simulink model "simulink_model_S"  (R2022a)
settings: Solver=VariableStepAuto  StartTime=0.0  StopTime=100  RelTol=1e-3
values from neighbouring files (symbols this model uses):
  b1 = 8    [Simulink_model_M.m]    (also in Stavovy_model_G1_M.m; Stavovy_model_G2_M.m)
  b2 = 1.6    [Simulink_model_M.m]    (also in Stavovy_model_G1_M.m; Stavovy_model_G2_M.m; Vysetrenie_vplyvu_zmeny_parametrov_G3.m = double(b2))
  F2 = 0    [Simulink_model_M.m]    (also in Stavovy_model_G1_M.m; Stavovy_model_G2_M.m)
  k1 = 400    [Simulink_model_M.m]    (also in Stavovy_model_G1_M.m; Stavovy_model_G2_M.m)
  k2 = 80    [Simulink_model_M.m]    (also in Stavovy_model_G1_M.m; Stavovy_model_G2_M.m)
  m1 = 0.5    [Simulink_model_M.m]    (also in Stavovy_model_G1_M.m; Stavovy_model_G2_M.m)
  m2 = 0.1    [Simulink_model_M.m]    (also in Stavovy_model_G1_M.m; Stavovy_model_G2_M.m)
settings Model: Creator=Ivan  LastModifiedBy=Ivan

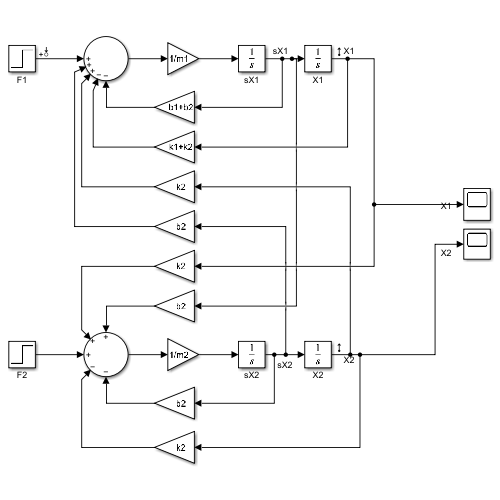
[thumbnail: Simulink's stored preview of the top-level diagram]
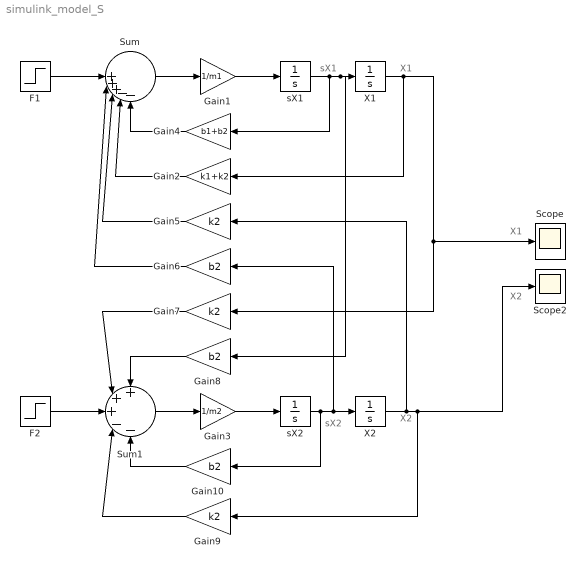
== system simulink_model_S ==
  note: X1
  note: X1
  note: sX1
  note: X2
  note: sX2
  note: X2
  F1 : Step  Time=0  After=10  SampleTime=0
  F2 : Step  Time=0  After=F2  SampleTime=0
  Gain1 : Gain  Gain=1/m1
  Gain10 : Gain  Gain=b2
  Gain2 : Gain  Gain=k1+k2
  Gain3 : Gain  Gain=1/m2
  Gain4 : Gain  Gain=b1+b2
  Gain5 : Gain  Gain=k2
  Gain6 : Gain  Gain=b2
  Gain7 : Gain  Gain=k2
  Gain8 : Gain  Gain=b2
  Gain9 : Gain  Gain=k2
  Scope : Scope
  Scope2 : Scope
  Sum : Sum  Inputs=||||+++--
  Sum1 : Sum  Inputs=+++--
  X1 : Integrator
  X2 : Integrator
  sX1 : Integrator
  sX2 : Integrator
  wires:
  sX1/1 -> Gain4/1, Gain8/1, X1/1
  X2/1 -> Gain5/1, Gain9/1, Scope2/1
  sX2/1 -> Gain10/1, Gain6/1, X2/1
  Gain1/1 -> sX1/1
  Sum/1 -> Gain1/1
  F1/1 -> Sum/1
  X1/1 -> Gain2/1, Gain7/1, Scope/1
  Gain2/1 -> Sum/4
  Gain4/1 -> Sum/5
  Sum1/1 -> Gain3/1
  Gain3/1 -> sX2/1
  F2/1 -> Sum1/3
  Gain5/1 -> Sum/3
  Gain6/1 -> Sum/2
  Gain7/1 -> Sum1/2
  Gain8/1 -> Sum1/1
  Gain10/1 -> Sum1/5
  Gain9/1 -> Sum1/4
